simulink model "bh_COMPONENT_1dof_NEWTON"  (R2026b)
settings: Solver=VariableStepAuto
model mask{m=plant_T.m, c=plant_T.c, k=plant_T.k, y0=IC_T.y, y_dot_0=IC_T.y_dot}
  mask prompts: m "m  (kg)"; c "c (N.s/m)"; k "k (N/m)"; y0 "y0 (m)"; y_dot_0 "y_dot_0  (m/s)"
settings Model: Creator=bhorton  LastModifiedBy=bhorton

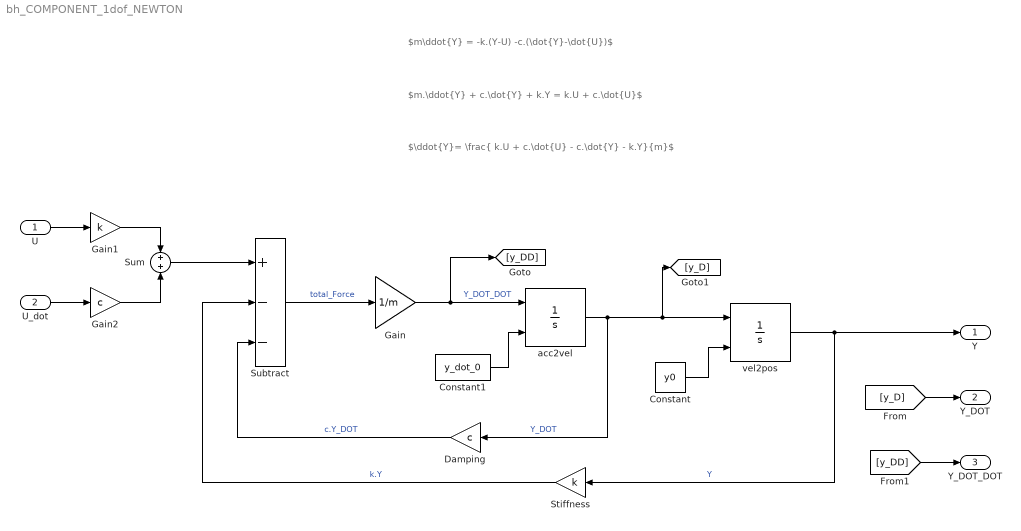
== system bh_COMPONENT_1dof_NEWTON ==
  note: $m.\ddot{Y} + c.\dot{Y} + k.Y = k.U + c.\dot{U}$
  note: $m\ddot{Y} = -k.(Y-U) -c.(\dot{Y}-\dot{U})$
  note: $\ddot{Y}= \frac{ k.U + c.\dot{U} - c.\dot{Y} - k.Y}{m}$
  U : Inport
  U_dot : Inport  Port=2
  Constant : Constant  Value=y0
  Constant1 : Constant  Value=y_dot_0
  Damping : Gain  Gain=c
  Gain : Gain  Gain=1/m
  Gain1 : Gain  Gain=k
  Gain2 : Gain  Gain=c
  Stiffness : Gain  Gain=k
  Subtract : Sum  Inputs=+--
  Sum : Sum  Inputs=+|+
  acc2vel : Integrator  InitialConditionSource=external
  vel2pos : Integrator  InitialConditionSource=external
  Y : Outport
  Y_DOT : Outport  Port=2
  Y_DOT_DOT : Outport  Port=3
  wires:
  Gain/1 -> acc2vel/1, [y_DD]  "Y_DOT_DOT"
  Constant1/1 -> acc2vel/2
  Stiffness/1 -> Subtract/2  "k.Y"
  vel2pos/1 -> Stiffness/1, Y/1  "Y"
  Subtract/1 -> Gain/1  "total_Force"
  Constant/1 -> vel2pos/2
  acc2vel/1 -> Damping/1, vel2pos/1, [y_D]  "Y_DOT"
  Damping/1 -> Subtract/3  "c.Y_DOT"
  [y_D] -> Y_DOT/1
  [y_DD] -> Y_DOT_DOT/1
  Sum/1 -> Subtract/1
  Gain2/1 -> Sum/2
  Gain1/1 -> Sum/1
  U/1 -> Gain1/1
  U_dot/1 -> Gain2/1
